simulink model "control_pmsm"  (R2024a)
settings: Solver=FixedStepAuto  StartTime=0.0  StopTime=100  RelTol=1e-3  EnableMultiTasking=on
undefined symbols (not defined in the file): ControlModes, EstimationVelocityModes, Ts_ControlFOC
settings Model: DataDictionary=EmbeddedBoardDD.sldd  Creator=upattacini  LastModifiedBy=mfussi
settings SolverCC: AllowMultiTaskInputOutput=on  AutoInsertRateTranBlk=on  InsertRTBMode=Never (minimum delay)
settings DataIOCC: SaveOutput=off  DSMLogging=off  SaveTime=off  ReturnWorkspaceOutputs=off
settings DebuggingCC: ParameterPrecisionLossMsg=none  UnconnectedInputMsg=warning  UnconnectedOutputMsg=warning  UnconnectedLineMsg=warning
settings ModelReferenceCC: EnableRefExpFcnMdlSchedulingChecks=on
settings RTWCC: GPUComputeCapability=3.5  DLArmComputeVersion=19.05

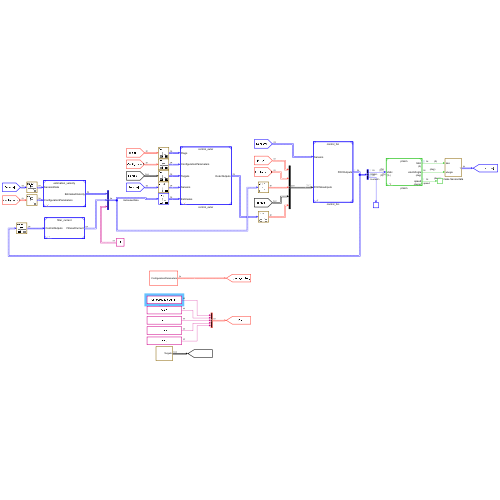
[thumbnail: Simulink's stored preview of the top-level diagram]
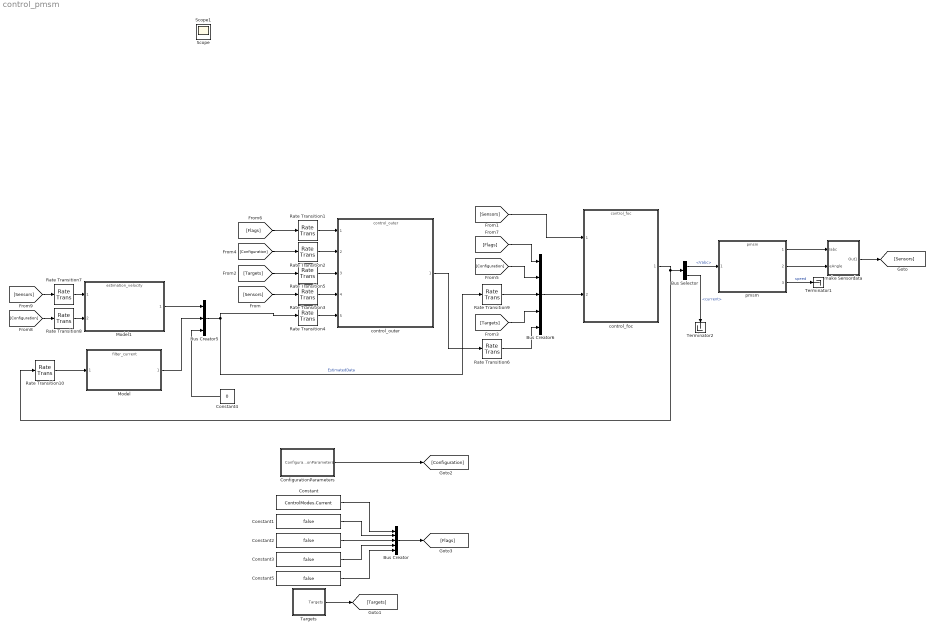
== system control_pmsm ==
  Bus Creator : BusCreator  Inputs=5  OutDataTypeStr=Bus: Flags  NonVirtualBus=on
      settings: InheritFromInputs=off
  Bus Creator5 : BusCreator  Inputs=3  OutDataTypeStr=Bus: EstimatedData  NonVirtualBus=on
      settings: InheritFromInputs=off
  Bus Creator6 : BusCreator  Inputs=5  OutDataTypeStr=Bus: FOCSlowInputs  NonVirtualBus=on
      settings: InheritFromInputs=off
  Bus Selector : BusSelector  OutputSignals=Vabc,Iq_fbk.current
  ConfigurationParameters : Subsystem
  Constant : Constant  Value=ControlModes.Current  OutDataTypeStr=Enum: ControlModes  LockScale=on
  Constant{1..3,5} (4 alike) : Constant  Value=false  OutDataTypeStr=boolean  LockScale=on
  Constant4 : Constant  Value=0  OutDataTypeStr=Bus: MotorTemperature
  Model : ModelReference  ModelNameDialog=filter_current.slx  SimulationMode=Normal  ModelReferenceVersion=6.3
  Model1 : ModelReference  ModelNameDialog=estimation_velocity.slx  SimulationMode=Normal  ModelReferenceVersion=6.4
  Rate Transition{1..5} (5 alike) : RateTransition  Deterministic=off  OutPortSampleTime=Ts_ControlOuter
  Rate Transition{6..10} (5 alike) : RateTransition  Deterministic=off
  Targets : Subsystem
  Terminator1 : Terminator
  Terminator2 : Terminator
  control_foc : ModelReference  ModelNameDialog=control_foc.slx  SimulationMode=Normal  ModelReferenceVersion=6.19
  control_outer : ModelReference  ModelNameDialog=control_outer.slx  SimulationMode=Normal  ModelReferenceVersion=6.3
  make Sensordata : Subsystem
  pmsm : ModelReference  ModelNameDialog=pmsm.slx  SimulationMode=Normal  ModelReferenceVersion=8.1
  Scope : Scope
  Scope1 : Scope
  wires:
  control_foc/1 -> Bus Selector/1, Rate Transition10/1
  Bus Selector/1 -> pmsm/1  "<Vabc>"
  Constant/1 -> Bus Creator/1
  pmsm/3 -> Terminator1/1  "speed"
  Targets/1(Targets) -> [Targets]
  ConfigurationParameters/1(ConfigurationParameters) -> [Configuration]
  Bus Creator/1 -> [Flags]
  [Flags] -> Rate Transition1/1
  Rate Transition1/1 -> control_outer/1
  Rate Transition2/1 -> control_outer/2
  [Configuration] -> Rate Transition2/1
  Rate Transition3/1 -> control_outer/4
  [Sensors] -> Rate Transition3/1
  Rate Transition4/1 -> control_outer/5
  Rate Transition5/1 -> control_outer/3
  [Targets] -> Rate Transition5/1
  control_outer/1 -> Rate Transition6/1
  Bus Creator6/1 -> control_foc/2
  [Targets] -> Bus Creator6/4
  Rate Transition6/1 -> Bus Creator6/5
  Bus Creator5/1 -> Rate Transition4/1, Rate Transition9/1  "EstimatedData"
  [Configuration] -> Bus Creator6/2
  [Flags] -> Bus Creator6/1
  [Sensors] -> control_foc/1
  Constant1/1 -> Bus Creator/2
  Constant2/1 -> Bus Creator/3
  Model1/1 -> Bus Creator5/1
  Model/1 -> Bus Creator5/2
  [Configuration] -> Rate Transition8/1
  [Sensors] -> Rate Transition7/1
  Rate Transition7/1 -> Model1/1
  Rate Transition8/1 -> Model1/2
  Rate Transition9/1 -> Bus Creator6/3
  Rate Transition10/1 -> Model/1
  Constant3/1 -> Bus Creator/4
  Constant4/1 -> Bus Creator5/3
  Constant5/1 -> Bus Creator/5
  pmsm/1 -> make Sensordata/1(Iabc)
  pmsm/2 -> make Sensordata/2(eAngle)
  make Sensordata/1(Out1) -> [Sensors]
  Bus Selector/2 -> Terminator2/1  "<current>"

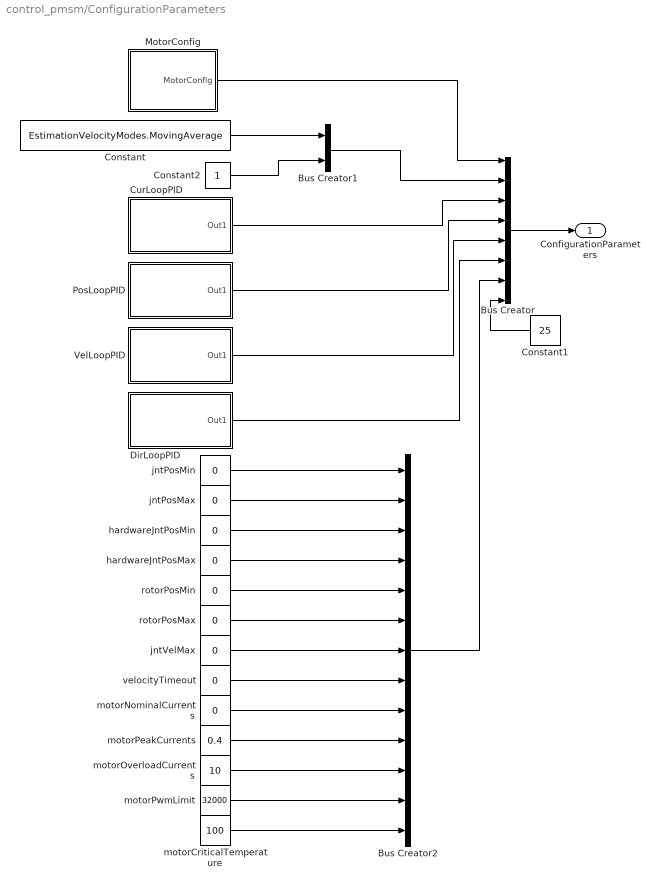
== system control_pmsm/ConfigurationParameters ==
  Bus Creator : BusCreator  Inputs=8  OutDataTypeStr=Bus: ConfigurationParameters  NonVirtualBus=on
      settings: InheritFromInputs=off
  Bus Creator1 : BusCreator  Inputs=2  OutDataTypeStr=Bus: EstimationConfig  NonVirtualBus=on
      settings: InheritFromInputs=off
  Bus Creator2 : BusCreator  Inputs=13  OutDataTypeStr=Bus: Thresholds  NonVirtualBus=on
      settings: InheritFromInputs=off
  Constant : Constant  Value=EstimationVelocityModes.MovingAverage  OutDataTypeStr=Enum: EstimationVelocityModes
  Constant1 : Constant  Value=25  OutDataTypeStr=single
  Constant2 : Constant  OutDataTypeStr=single
  CurLoopPID : Subsystem  mask{OutMax=0, OutMin=0, P=2, I=500, D=0, N=10, I0=0, D0=0, shift_factor=0}
      mask prompts: shift_factor "Shift Factor"
  DirLoopPID : Subsystem  mask{OutMax=0, OutMin=0, P=0, I=0, D=0, N=0, I0=0, D0=0, shift_factor=0}
      mask prompts: shift_factor "Shift Factor"
  MotorConfig : Subsystem  mask{hall_sens_offset=30, has_hall_sens=true, has_quadrature_encoder=true, has_speed_quadrature_encoder=false, has_torque_sens=false, use_index=true, enable_verbosity=false, rotor_encoder_resolution=16000, rotor_index_offset=0, encoder_tolerance=0, pole_pairs=7, reduction=1, Kbemf=0, Rphase=0, Imin=-10, Imax=10, Vmax=24, R=29.5, L=200, Rt=50, tau=200}
      mask prompts: R "Motor Resistance"; L "Motor Inductance"; Rt "Thermal Resistance"; tau "Thermal Time Constant"
  PosLoopPID : Subsystem  mask{OutMax=0, OutMin=0, P=0, I=0, D=0, N=0, I0=0, D0=0, shift_factor=0}
      mask prompts: shift_factor "Shift Factor"
  VelLoopPID : Subsystem  mask{OutMax=0, OutMin=0, P=0, I=0, D=0, N=0, I0=0, D0=0, shift_factor=0}
      mask prompts: shift_factor "Shift Factor"
  hardwareJntPosMax : Constant  Value=0  OutDataTypeStr=single
  hardwareJntPosMin : Constant  Value=0  OutDataTypeStr=single
  jntPosMax : Constant  Value=0  OutDataTypeStr=single
  jntPosMin : Constant  Value=0  OutDataTypeStr=single
  jntVelMax : Constant  Value=0  OutDataTypeStr=single
  motorCriticalTemperature : Constant  Value=100  OutDataTypeStr=single
  motorNominalCurrents : Constant  Value=0  OutDataTypeStr=single
  motorOverloadCurrents : Constant  Value=10  OutDataTypeStr=single
  motorPeakCurrents : Constant  Value=0.4  OutDataTypeStr=single
  motorPwmLimit : Constant  Value=32000  OutDataTypeStr=uint32
  rotorPosMax : Constant  Value=0  OutDataTypeStr=single
  rotorPosMin : Constant  Value=0  OutDataTypeStr=single
  velocityTimeout : Constant  Value=0  OutDataTypeStr=uint32
  ConfigurationParameters : Outport
  wires:
  Bus Creator/1 -> ConfigurationParameters/1
  Constant/1 -> Bus Creator1/1
  jntPosMin/1 -> Bus Creator2/1
  jntPosMax/1 -> Bus Creator2/2
  hardwareJntPosMin/1 -> Bus Creator2/3
  hardwareJntPosMax/1 -> Bus Creator2/4
  rotorPosMin/1 -> Bus Creator2/5
  rotorPosMax/1 -> Bus Creator2/6
  jntVelMax/1 -> Bus Creator2/7
  velocityTimeout/1 -> Bus Creator2/8
  motorNominalCurrents/1 -> Bus Creator2/9
  motorPeakCurrents/1 -> Bus Creator2/10
  motorOverloadCurrents/1 -> Bus Creator2/11
  motorPwmLimit/1 -> Bus Creator2/12
  Bus Creator1/1 -> Bus Creator/2
  PosLoopPID/1(Out1) -> Bus Creator/4
  CurLoopPID/1(Out1) -> Bus Creator/3
  VelLoopPID/1(Out1) -> Bus Creator/5
  MotorConfig/1(MotorConfig) -> Bus Creator/1
  DirLoopPID/1(Out1) -> Bus Creator/6
  Bus Creator2/1 -> Bus Creator/7
  Constant1/1 -> Bus Creator/8
  motorCriticalTemperature/1 -> Bus Creator2/13
  Constant2/1 -> Bus Creator1/2

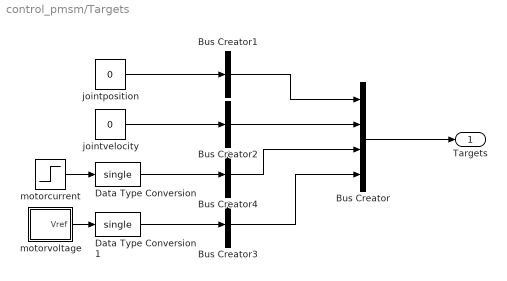
== system control_pmsm/Targets ==
  Bus Creator : BusCreator  Inputs=4  OutDataTypeStr=Bus: Targets  NonVirtualBus=on
      settings: InheritFromInputs=off
  Bus Creator1 : BusCreator  Inputs=1  OutDataTypeStr=Bus: JointPositions  NonVirtualBus=on
      settings: InheritFromInputs=off
  Bus Creator2 : BusCreator  Inputs=1  OutDataTypeStr=Bus: JointVelocities  NonVirtualBus=on
      settings: InheritFromInputs=off
  Bus Creator3 : BusCreator  Inputs=1  OutDataTypeStr=Bus: MotorVoltage  NonVirtualBus=on
      settings: InheritFromInputs=off
  Bus Creator4 : BusCreator  Inputs=1  OutDataTypeStr=Bus: MotorCurrent  NonVirtualBus=on
      settings: InheritFromInputs=off
  Data Type Conversion : DataTypeConversion  OutDataTypeStr=single  SaturateOnIntegerOverflow=off  RndMeth=Floor
  Data Type Conversion1 : DataTypeConversion  OutDataTypeStr=single  SaturateOnIntegerOverflow=off  RndMeth=Floor
  jointposition : Constant  Value=0  OutDataTypeStr=single
  jointvelocity : Constant  Value=0  OutDataTypeStr=single
  motorcurrent : Step  Time=0.1  After=0.8  SampleTime=0
  motorvoltage : Subsystem
  Targets : Outport
  wires:
  Bus Creator/1 -> Targets/1
  jointposition/1 -> Bus Creator1/1
  Bus Creator1/1 -> Bus Creator/1
  Bus Creator2/1 -> Bus Creator/2
  Bus Creator3/1 -> Bus Creator/4
  Bus Creator4/1 -> Bus Creator/3
  jointvelocity/1 -> Bus Creator2/1
  motorcurrent/1 -> Data Type Conversion/1
  Data Type Conversion1/1 -> Bus Creator3/1
  Data Type Conversion/1 -> Bus Creator4/1
  motorvoltage/1(Vref) -> Data Type Conversion1/1

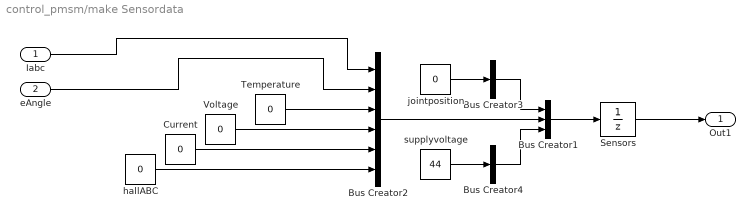
== system control_pmsm/make Sensordata ==
  Iabc : Inport
  eAngle : Inport  Port=2
  Bus Creator1 : BusCreator  Inputs=3  OutDataTypeStr=Bus: SensorsData  NonVirtualBus=on
      settings: InheritFromInputs=off
  Bus Creator2 : BusCreator  Inputs=6  OutDataTypeStr=Bus: MotorSensors  NonVirtualBus=on
      settings: InheritFromInputs=off
  Bus Creator3 : BusCreator  Inputs=1  OutDataTypeStr=Bus: JointPositions  NonVirtualBus=on
      settings: InheritFromInputs=off
  Bus Creator4 : BusCreator  Inputs=1  OutDataTypeStr=Bus: SupplyVoltage  NonVirtualBus=on
      settings: InheritFromInputs=off
  Current : Constant  Value=0  OutDataTypeStr=single  SampleTime=1e-5
  Sensors : UnitDelay  SampleTime=Ts_ControlFOC  HasFrameUpgradeWarning=on
  Temperature : Constant  Value=0  OutDataTypeStr=single  SampleTime=1e-5
  Voltage : Constant  Value=0  OutDataTypeStr=single  SampleTime=1e-5
  hallABC : Constant  Value=0  OutDataTypeStr=uint8  SampleTime=1e-5
  jointposition : Constant  Value=0  OutDataTypeStr=single  SampleTime=1e-5
  supplyvoltage : Constant  Value=44  OutDataTypeStr=single  SampleTime=1e-5
  Out1 : Outport
  wires:
  Voltage/1 -> Bus Creator2/4
  Bus Creator2/1 -> Bus Creator1/2
  Bus Creator1/1 -> Sensors/1
  jointposition/1 -> Bus Creator3/1
  Current/1 -> Bus Creator2/5
  Temperature/1 -> Bus Creator2/3
  supplyvoltage/1 -> Bus Creator4/1
  hallABC/1 -> Bus Creator2/6
  Bus Creator3/1 -> Bus Creator1/1
  Bus Creator4/1 -> Bus Creator1/3
  eAngle/1 -> Bus Creator2/2
  Sensors/1 -> Out1/1
  Iabc/1 -> Bus Creator2/1

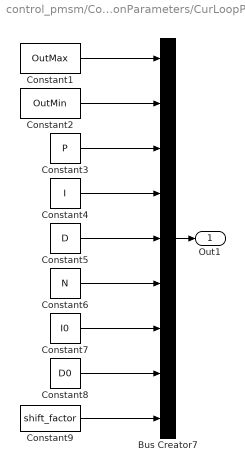
== system control_pmsm/ConfigurationParameters/CurLoopPID ==
  Bus Creator7 : BusCreator  Inputs=9  OutDataTypeStr=Bus: PIDConfig  NonVirtualBus=on
      settings: InheritFromInputs=off
  Constant1 : Constant  Value=OutMax  OutDataTypeStr=single
  Constant2 : Constant  Value=OutMin  OutDataTypeStr=single
  Constant3 : Constant  Value=P  OutDataTypeStr=single
  Constant4 : Constant  Value=I  OutDataTypeStr=single
  Constant5 : Constant  Value=D  OutDataTypeStr=single
  Constant6 : Constant  Value=N  OutDataTypeStr=single
  Constant7 : Constant  Value=I0  OutDataTypeStr=single
  Constant8 : Constant  Value=D0  OutDataTypeStr=single
  Constant9 : Constant  Value=shift_factor  OutDataTypeStr=uint8
  Out1 : Outport
  wires:
  Constant9/1 -> Bus Creator7/9
  Constant5/1 -> Bus Creator7/5
  Bus Creator7/1 -> Out1/1
  Constant8/1 -> Bus Creator7/8
  Constant2/1 -> Bus Creator7/2
  Constant4/1 -> Bus Creator7/4
  Constant7/1 -> Bus Creator7/7
  Constant1/1 -> Bus Creator7/1
  Constant3/1 -> Bus Creator7/3
  Constant6/1 -> Bus Creator7/6

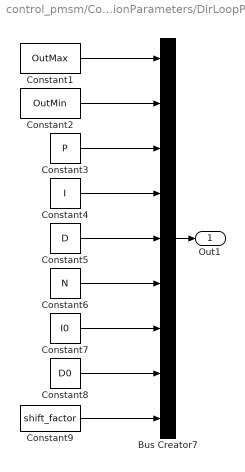
== system control_pmsm/ConfigurationParameters/DirLoopPID ==
  Bus Creator7 : BusCreator  Inputs=9  OutDataTypeStr=Bus: PIDConfig  NonVirtualBus=on
      settings: InheritFromInputs=off
  Constant1 : Constant  Value=OutMax  OutDataTypeStr=single
  Constant2 : Constant  Value=OutMin  OutDataTypeStr=single
  Constant3 : Constant  Value=P  OutDataTypeStr=single
  Constant4 : Constant  Value=I  OutDataTypeStr=single
  Constant5 : Constant  Value=D  OutDataTypeStr=single
  Constant6 : Constant  Value=N  OutDataTypeStr=single
  Constant7 : Constant  Value=I0  OutDataTypeStr=single
  Constant8 : Constant  Value=D0  OutDataTypeStr=single
  Constant9 : Constant  Value=shift_factor  OutDataTypeStr=uint8
  Out1 : Outport
  wires:
  Constant6/1 -> Bus Creator7/6
  Constant3/1 -> Bus Creator7/3
  Constant1/1 -> Bus Creator7/1
  Constant7/1 -> Bus Creator7/7
  Constant4/1 -> Bus Creator7/4
  Constant2/1 -> Bus Creator7/2
  Constant8/1 -> Bus Creator7/8
  Bus Creator7/1 -> Out1/1
  Constant5/1 -> Bus Creator7/5
  Constant9/1 -> Bus Creator7/9

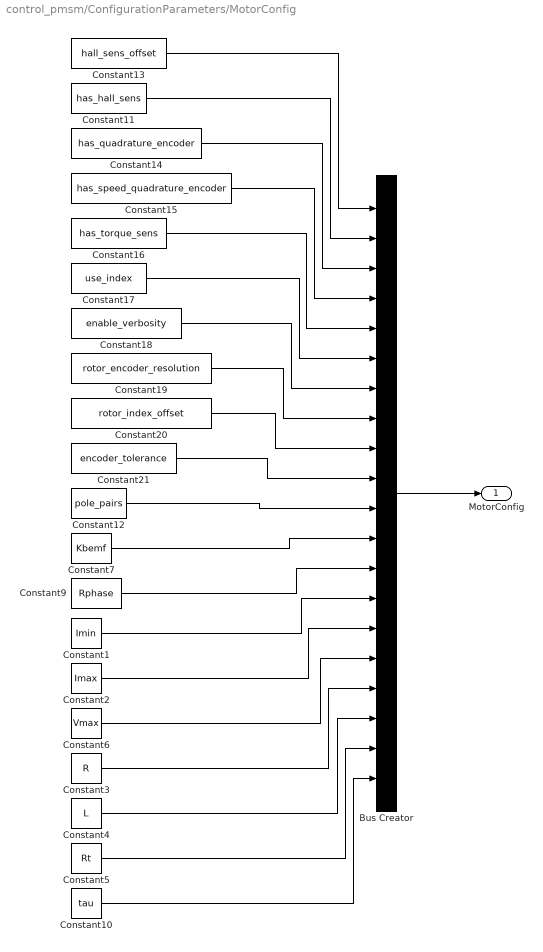
== system control_pmsm/ConfigurationParameters/MotorConfig ==
  Bus Creator : BusCreator  Inputs=20  OutDataTypeStr=Bus: MotorConfig  NonVirtualBus=on
      settings: InheritFromInputs=off
  Constant1 : Constant  Value=Imin  OutDataTypeStr=single
  Constant10 : Constant  Value=tau  OutDataTypeStr=single
  Constant11 : Constant  Value=has_hall_sens  OutDataTypeStr=boolean
  Constant12 : Constant  Value=pole_pairs  OutDataTypeStr=uint8
  Constant13 : Constant  Value=hall_sens_offset  OutDataTypeStr=single
  Constant14 : Constant  Value=has_quadrature_encoder  OutDataTypeStr=boolean
  Constant15 : Constant  Value=has_speed_quadrature_encoder  OutDataTypeStr=boolean
  Constant16 : Constant  Value=has_torque_sens  OutDataTypeStr=boolean
  Constant17 : Constant  Value=use_index  OutDataTypeStr=boolean
  Constant18 : Constant  Value=enable_verbosity  OutDataTypeStr=boolean
  Constant19 : Constant  Value=rotor_encoder_resolution  OutDataTypeStr=int16
  Constant2 : Constant  Value=Imax  OutDataTypeStr=single
  Constant20 : Constant  Value=rotor_index_offset  OutDataTypeStr=int16
  Constant21 : Constant  Value=encoder_tolerance  OutDataTypeStr=uint8
  Constant3 : Constant  Value=R  OutDataTypeStr=single
  Constant4 : Constant  Value=L  OutDataTypeStr=single
  Constant5 : Constant  Value=Rt  OutDataTypeStr=single
  Constant6 : Constant  Value=Vmax  OutDataTypeStr=single
  Constant7 : Constant  Value=Kbemf  OutDataTypeStr=single
  Constant9 : Constant  Value=Rphase  OutDataTypeStr=single
  MotorConfig : Outport
  wires:
  Bus Creator/1 -> MotorConfig/1
  Constant20/1 -> Bus Creator/9
  Constant19/1 -> Bus Creator/8
  Constant21/1 -> Bus Creator/10
  Constant15/1 -> Bus Creator/4
  Constant18/1 -> Bus Creator/7
  Constant12/1 -> Bus Creator/11
  Constant14/1 -> Bus Creator/3
  Constant16/1 -> Bus Creator/5
  Constant7/1 -> Bus Creator/12
  Constant17/1 -> Bus Creator/6
  Constant9/1 -> Bus Creator/13
  Constant1/1 -> Bus Creator/14
  Constant2/1 -> Bus Creator/15
  Constant13/1 -> Bus Creator/1
  Constant11/1 -> Bus Creator/2
  Constant6/1 -> Bus Creator/16
  Constant3/1 -> Bus Creator/17
  Constant4/1 -> Bus Creator/18
  Constant5/1 -> Bus Creator/19
  Constant10/1 -> Bus Creator/20

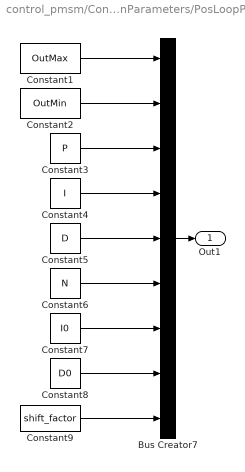
== system control_pmsm/ConfigurationParameters/PosLoopPID ==
  Bus Creator7 : BusCreator  Inputs=9  OutDataTypeStr=Bus: PIDConfig  NonVirtualBus=on
      settings: InheritFromInputs=off
  Constant1 : Constant  Value=OutMax  OutDataTypeStr=single
  Constant2 : Constant  Value=OutMin  OutDataTypeStr=single
  Constant3 : Constant  Value=P  OutDataTypeStr=single
  Constant4 : Constant  Value=I  OutDataTypeStr=single
  Constant5 : Constant  Value=D  OutDataTypeStr=single
  Constant6 : Constant  Value=N  OutDataTypeStr=single
  Constant7 : Constant  Value=I0  OutDataTypeStr=single
  Constant8 : Constant  Value=D0  OutDataTypeStr=single
  Constant9 : Constant  Value=shift_factor  OutDataTypeStr=uint8
  Out1 : Outport
  wires:
  Constant6/1 -> Bus Creator7/6
  Constant3/1 -> Bus Creator7/3
  Constant1/1 -> Bus Creator7/1
  Constant7/1 -> Bus Creator7/7
  Constant4/1 -> Bus Creator7/4
  Constant2/1 -> Bus Creator7/2
  Constant8/1 -> Bus Creator7/8
  Bus Creator7/1 -> Out1/1
  Constant5/1 -> Bus Creator7/5
  Constant9/1 -> Bus Creator7/9

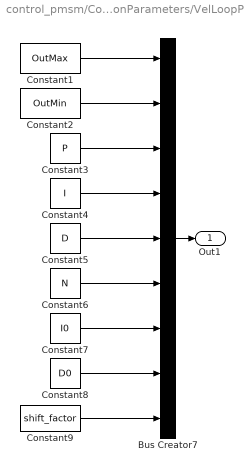
== system control_pmsm/ConfigurationParameters/VelLoopPID ==
  Bus Creator7 : BusCreator  Inputs=9  OutDataTypeStr=Bus: PIDConfig  NonVirtualBus=on
      settings: InheritFromInputs=off
  Constant1 : Constant  Value=OutMax  OutDataTypeStr=single
  Constant2 : Constant  Value=OutMin  OutDataTypeStr=single
  Constant3 : Constant  Value=P  OutDataTypeStr=single
  Constant4 : Constant  Value=I  OutDataTypeStr=single
  Constant5 : Constant  Value=D  OutDataTypeStr=single
  Constant6 : Constant  Value=N  OutDataTypeStr=single
  Constant7 : Constant  Value=I0  OutDataTypeStr=single
  Constant8 : Constant  Value=D0  OutDataTypeStr=single
  Constant9 : Constant  Value=shift_factor  OutDataTypeStr=uint8
  Out1 : Outport
  wires:
  Constant9/1 -> Bus Creator7/9
  Constant5/1 -> Bus Creator7/5
  Bus Creator7/1 -> Out1/1
  Constant8/1 -> Bus Creator7/8
  Constant2/1 -> Bus Creator7/2
  Constant4/1 -> Bus Creator7/4
  Constant7/1 -> Bus Creator7/7
  Constant1/1 -> Bus Creator7/1
  Constant3/1 -> Bus Creator7/3
  Constant6/1 -> Bus Creator7/6

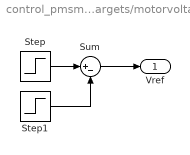
== system control_pmsm/Targets/motorvoltage ==
  Step : Step  Time=0.1  After=100  SampleTime=0
  Step1 : Step  Time=0.2  After=60  SampleTime=0
  Sum : Sum  Inputs=|+-
  Vref : Outport
  wires:
  Sum/1 -> Vref/1
  Step1/1 -> Sum/2
  Step/1 -> Sum/1
